simulink model "SuspensionModelBase"  (R2025b)
settings: Solver=ode23t  StartTime=0.0  StopTime=5  RelTol=1e-3
values from neighbouring files (symbols this model uses):
  car = get_suspension_default_params()    [run_suspension_standalone.m]
settings Model: Creator=91984  LastModifiedBy=91984

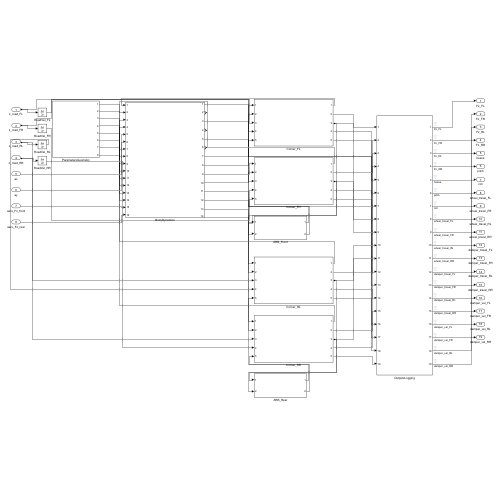
[thumbnail: Simulink's stored preview of the top-level diagram]
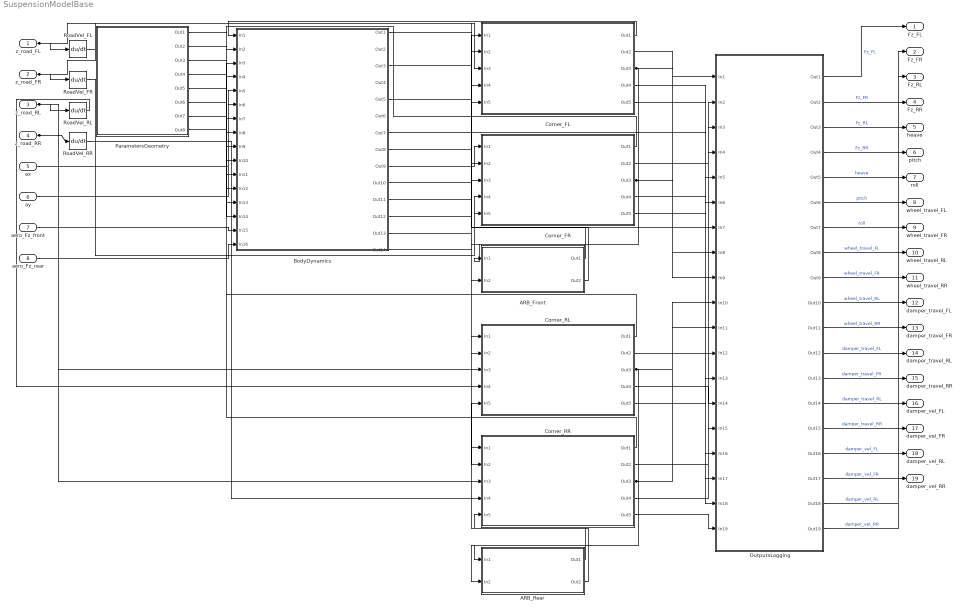
== system SuspensionModelBase ==
  z_road_FL : Inport
  z_road_FR : Inport  Port=2
  z_road_RL : Inport  Port=3
  z_road_RR : Inport  Port=4
  ax : Inport  Port=5
  ay : Inport  Port=6
  aero_Fz_front : Inport  Port=7
  aero_Fz_rear : Inport  Port=8
  ARB_Front : Subsystem
  ARB_Rear : Subsystem
  BodyDynamics : Subsystem
  Corner_FL : Subsystem
  Corner_FR : Subsystem
  Corner_RL : Subsystem
  Corner_RR : Subsystem
  OutputsLogging : Subsystem
  ParametersGeometry : Subsystem
  RoadVel_FL : Derivative
  RoadVel_FR : Derivative
  RoadVel_RL : Derivative
  RoadVel_RR : Derivative
  Fz_FL : Outport
  Fz_FR : Outport  Port=2
  Fz_RL : Outport  Port=3
  Fz_RR : Outport  Port=4
  heave : Outport  Port=5
  pitch : Outport  Port=6
  roll : Outport  Port=7
  wheel_travel_FL : Outport  Port=8
  wheel_travel_FR : Outport  Port=9
  wheel_travel_RL : Outport  Port=10
  wheel_travel_RR : Outport  Port=11
  damper_travel_FL : Outport  Port=12
  damper_travel_FR : Outport  Port=13
  damper_travel_RL : Outport  Port=14
  damper_travel_RR : Outport  Port=15
  damper_vel_FL : Outport  Port=16
  damper_vel_FR : Outport  Port=17
  damper_vel_RL : Outport  Port=18
  damper_vel_RR : Outport  Port=19
  wires:
  z_road_FL/1 -> RoadVel_FL/1, Corner_FL/3(In3)
  RoadVel_FL/1 -> Corner_FL/4(In4)
  z_road_FR/1 -> RoadVel_FR/1, Corner_FR/3(In3)
  RoadVel_FR/1 -> Corner_FR/4(In4)
  z_road_RL/1 -> RoadVel_RL/1, Corner_RL/3(In3)
  RoadVel_RL/1 -> Corner_RL/4(In4)
  z_road_RR/1 -> RoadVel_RR/1, Corner_RR/3(In3)
  RoadVel_RR/1 -> Corner_RR/4(In4)
  ax/1 -> BodyDynamics/5(In5)
  ay/1 -> BodyDynamics/6(In6)
  aero_Fz_front/1 -> BodyDynamics/15(In15)
  aero_Fz_rear/1 -> BodyDynamics/16(In16)
  ParametersGeometry/1(Out1) -> BodyDynamics/7(In7)
  ParametersGeometry/2(Out2) -> BodyDynamics/8(In8)
  ParametersGeometry/3(Out3) -> BodyDynamics/9(In9)
  ParametersGeometry/4(Out4) -> BodyDynamics/10(In10)
  ParametersGeometry/5(Out5) -> BodyDynamics/11(In11)
  ParametersGeometry/6(Out6) -> BodyDynamics/12(In12)
  ParametersGeometry/7(Out7) -> BodyDynamics/13(In13)
  ParametersGeometry/8(Out8) -> BodyDynamics/14(In14)
  BodyDynamics/7(Out7) -> Corner_FL/1(In1)
  BodyDynamics/8(Out8) -> Corner_FL/2(In2)
  BodyDynamics/9(Out9) -> Corner_FR/1(In1)
  BodyDynamics/10(Out10) -> Corner_FR/2(In2)
  BodyDynamics/11(Out11) -> Corner_RL/1(In1)
  BodyDynamics/12(Out12) -> Corner_RL/2(In2)
  BodyDynamics/13(Out13) -> Corner_RR/1(In1)
  BodyDynamics/14(Out14) -> Corner_RR/2(In2)
  Corner_FL/1(Out1) -> BodyDynamics/1(In1)
  Corner_FR/1(Out1) -> BodyDynamics/2(In2)
  Corner_RL/1(Out1) -> BodyDynamics/3(In3)
  Corner_RR/1(Out1) -> BodyDynamics/4(In4)
  Corner_FL/3(Out3) -> ARB_Front/1(In1), OutputsLogging/8(In8)
  Corner_FR/3(Out3) -> ARB_Front/2(In2), OutputsLogging/9(In9)
  ARB_Front/1(Out1) -> Corner_FL/5(In5)
  ARB_Front/2(Out2) -> Corner_FR/5(In5)
  Corner_RL/3(Out3) -> ARB_Rear/1(In1), OutputsLogging/10(In10)
  Corner_RR/3(Out3) -> ARB_Rear/2(In2), OutputsLogging/11(In11)
  ARB_Rear/1(Out1) -> Corner_RL/5(In5)
  ARB_Rear/2(Out2) -> Corner_RR/5(In5)
  Corner_FL/2(Out2) -> OutputsLogging/1(In1)
  Corner_FR/2(Out2) -> OutputsLogging/2(In2)
  Corner_RL/2(Out2) -> OutputsLogging/3(In3)
  Corner_RR/2(Out2) -> OutputsLogging/4(In4)
  BodyDynamics/1(Out1) -> OutputsLogging/5(In5)
  BodyDynamics/3(Out3) -> OutputsLogging/6(In6)
  BodyDynamics/5(Out5) -> OutputsLogging/7(In7)
  Corner_FL/4(Out4) -> OutputsLogging/12(In12)
  Corner_FR/4(Out4) -> OutputsLogging/13(In13)
  Corner_RL/4(Out4) -> OutputsLogging/14(In14)
  Corner_RR/4(Out4) -> OutputsLogging/15(In15)
  Corner_FL/5(Out5) -> OutputsLogging/16(In16)
  Corner_FR/5(Out5) -> OutputsLogging/17(In17)
  Corner_RL/5(Out5) -> OutputsLogging/18(In18)
  Corner_RR/5(Out5) -> OutputsLogging/19(In19)
  OutputsLogging/1(Out1) -> Fz_FL/1  "Fz_FL"
  OutputsLogging/2(Out2) -> Fz_FR/1  "Fz_FR"
  OutputsLogging/3(Out3) -> Fz_RL/1  "Fz_RL"
  OutputsLogging/4(Out4) -> Fz_RR/1  "Fz_RR"
  OutputsLogging/5(Out5) -> heave/1  "heave"
  OutputsLogging/6(Out6) -> pitch/1  "pitch"
  OutputsLogging/7(Out7) -> roll/1  "roll"
  OutputsLogging/8(Out8) -> wheel_travel_FL/1  "wheel_travel_FL"
  OutputsLogging/9(Out9) -> wheel_travel_FR/1  "wheel_travel_FR"
  OutputsLogging/10(Out10) -> wheel_travel_RL/1  "wheel_travel_RL"
  OutputsLogging/11(Out11) -> wheel_travel_RR/1  "wheel_travel_RR"
  OutputsLogging/12(Out12) -> damper_travel_FL/1  "damper_travel_FL"
  OutputsLogging/13(Out13) -> damper_travel_FR/1  "damper_travel_FR"
  OutputsLogging/14(Out14) -> damper_travel_RL/1  "damper_travel_RL"
  OutputsLogging/15(Out15) -> damper_travel_RR/1  "damper_travel_RR"
  OutputsLogging/16(Out16) -> damper_vel_FL/1  "damper_vel_FL"
  OutputsLogging/17(Out17) -> damper_vel_FR/1  "damper_vel_FR"
  OutputsLogging/18(Out18) -> damper_vel_RL/1  "damper_vel_RL"
  OutputsLogging/19(Out19) -> damper_vel_RR/1  "damper_vel_RR"

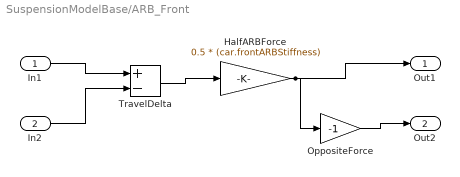
== system SuspensionModelBase/ARB_Front ==
  In1 : Inport
  In2 : Inport  Port=2
  HalfARBForce : Gain  Gain=0.5 * (car.frontARBStiffness)
  OppositeForce : Gain  Gain=-1
  TravelDelta : Sum  Inputs=+-
  Out1 : Outport
  Out2 : Outport  Port=2
  wires:
  In1/1 -> TravelDelta/1
  In2/1 -> TravelDelta/2
  TravelDelta/1 -> HalfARBForce/1
  HalfARBForce/1 -> Out1/1, OppositeForce/1
  OppositeForce/1 -> Out2/1

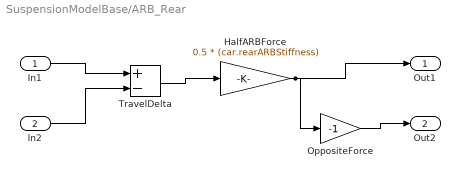
== system SuspensionModelBase/ARB_Rear ==
  In1 : Inport
  In2 : Inport  Port=2
  HalfARBForce : Gain  Gain=0.5 * (car.rearARBStiffness)
  OppositeForce : Gain  Gain=-1
  TravelDelta : Sum  Inputs=+-
  Out1 : Outport
  Out2 : Outport  Port=2
  wires:
  In1/1 -> TravelDelta/1
  In2/1 -> TravelDelta/2
  TravelDelta/1 -> HalfARBForce/1
  HalfARBForce/1 -> Out1/1, OppositeForce/1
  OppositeForce/1 -> Out2/1

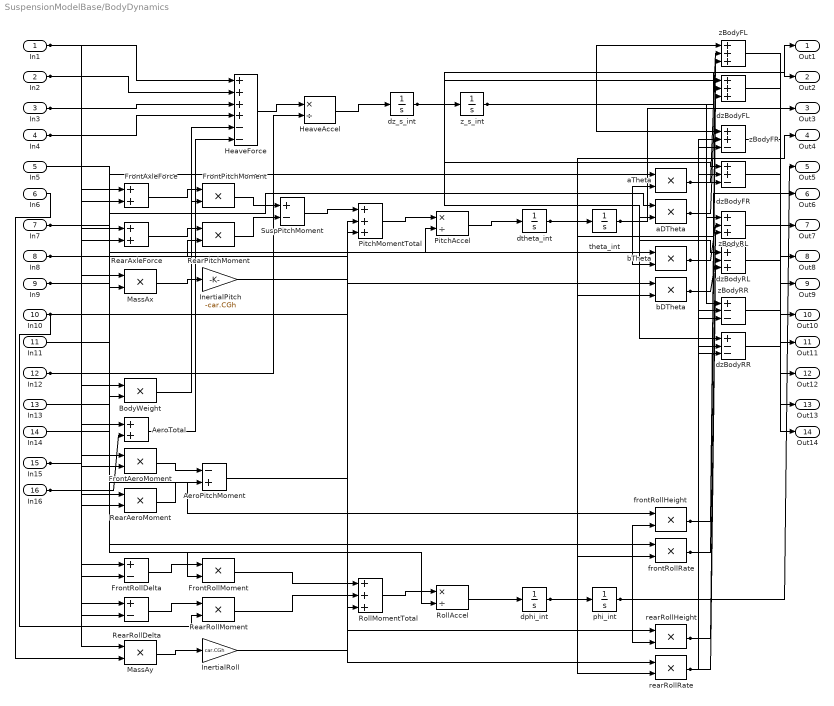
== system SuspensionModelBase/BodyDynamics ==
  In1 : Inport
  In2 : Inport  Port=2
  In3 : Inport  Port=3
  In4 : Inport  Port=4
  In5 : Inport  Port=5
  In6 : Inport  Port=6
  In7 : Inport  Port=7
  In8 : Inport  Port=8
  In9 : Inport  Port=9
  In10 : Inport  Port=10
  In11 : Inport  Port=11
  In12 : Inport  Port=12
  In13 : Inport  Port=13
  In14 : Inport  Port=14
  In15 : Inport  Port=15
  In16 : Inport  Port=16
  AeroPitchMoment : Sum  Inputs=-+
  AeroTotal : Sum
  BodyWeight : Product  Inputs=**
  FrontAeroMoment : Product  Inputs=**
  FrontAxleForce : Sum
  FrontPitchMoment : Product  Inputs=**
  FrontRollDelta : Sum  Inputs=+-
  FrontRollMoment : Product  Inputs=**
  HeaveAccel : Product  Inputs=*/
  HeaveForce : Sum  Inputs=++++--
  InertialPitch : Gain  Gain=-car.CGh
  InertialRoll : Gain  Gain=car.CGh
  MassAx : Product  Inputs=**
  MassAy : Product  Inputs=**
  PitchAccel : Product  Inputs=*/
  PitchMomentTotal : Sum  Inputs=+++
  RearAeroMoment : Product  Inputs=**
  RearAxleForce : Sum
  RearPitchMoment : Product  Inputs=**
  RearRollDelta : Sum  Inputs=+-
  RearRollMoment : Product  Inputs=**
  RollAccel : Product  Inputs=*/
  RollMomentTotal : Sum  Inputs=+++
  SuspPitchMoment : Sum  Inputs=+-
  aDTheta : Product  Inputs=**
  aTheta : Product  Inputs=**
  bDTheta : Product  Inputs=**
  bTheta : Product  Inputs=**
  dphi_int : Integrator
  dtheta_int : Integrator
  dzBodyFL : Sum  Inputs=+++
  dzBodyFR : Sum  Inputs=++-
  dzBodyRL : Sum  Inputs=+-+
  dzBodyRR : Sum  Inputs=+--
  dz_s_int : Integrator
  frontRollHeight : Product  Inputs=**
  frontRollRate : Product  Inputs=**
  phi_int : Integrator
  rearRollHeight : Product  Inputs=**
  rearRollRate : Product  Inputs=**
  theta_int : Integrator
  zBodyFL : Sum  Inputs=+++
  zBodyFR : Sum  Inputs=++-
  zBodyRL : Sum  Inputs=+-+
  zBodyRR : Sum  Inputs=+--
  z_s_int : Integrator
  Out1 : Outport
  Out2 : Outport  Port=2
  Out3 : Outport  Port=3
  Out4 : Outport  Port=4
  Out5 : Outport  Port=5
  Out6 : Outport  Port=6
  Out7 : Outport  Port=7
  Out8 : Outport  Port=8
  Out9 : Outport  Port=9
  Out10 : Outport  Port=10
  Out11 : Outport  Port=11
  Out12 : Outport  Port=12
  Out13 : Outport  Port=13
  Out14 : Outport  Port=14
  wires:
  In1/1 -> HeaveForce/1, FrontAxleForce/1, FrontRollDelta/1
  In2/1 -> HeaveForce/2, FrontAxleForce/2, FrontRollDelta/2
  In3/1 -> HeaveForce/3, RearAxleForce/1, RearRollDelta/1
  In4/1 -> HeaveForce/4, RearAxleForce/2, RearRollDelta/2
  In12/1 -> BodyWeight/1, HeaveAccel/2, MassAx/1, MassAy/1
  In11/1 -> BodyWeight/2
  BodyWeight/1 -> HeaveForce/5
  In15/1 -> AeroTotal/1, FrontAeroMoment/1
  In16/1 -> AeroTotal/2, RearAeroMoment/1
  AeroTotal/1 -> HeaveForce/6
  HeaveForce/1 -> HeaveAccel/1
  HeaveAccel/1 -> dz_s_int/1
  dz_s_int/1 -> z_s_int/1, Out2/1, dzBodyFL/1, dzBodyFR/1, dzBodyRL/1, dzBodyRR/1
  z_s_int/1 -> Out1/1, zBodyFL/1, zBodyFR/1, zBodyRL/1, zBodyRR/1
  FrontAxleForce/1 -> FrontPitchMoment/1
  In7/1 -> FrontPitchMoment/2, FrontAeroMoment/2, aTheta/1, aDTheta/1
  RearAxleForce/1 -> RearPitchMoment/1
  In8/1 -> RearPitchMoment/2, RearAeroMoment/2, bTheta/1, bDTheta/1
  FrontPitchMoment/1 -> SuspPitchMoment/1
  RearPitchMoment/1 -> SuspPitchMoment/2
  In5/1 -> MassAx/2
  MassAx/1 -> InertialPitch/1
  FrontAeroMoment/1 -> AeroPitchMoment/1
  RearAeroMoment/1 -> AeroPitchMoment/2
  SuspPitchMoment/1 -> PitchMomentTotal/1
  InertialPitch/1 -> PitchMomentTotal/2
  AeroPitchMoment/1 -> PitchMomentTotal/3
  PitchMomentTotal/1 -> PitchAccel/1
  In13/1 -> PitchAccel/2
  PitchAccel/1 -> dtheta_int/1
  dtheta_int/1 -> theta_int/1, Out4/1, aDTheta/2, bDTheta/2
  theta_int/1 -> Out3/1, aTheta/2, bTheta/2
  FrontRollDelta/1 -> FrontRollMoment/1
  In9/1 -> FrontRollMoment/2, frontRollHeight/1, frontRollRate/1
  RearRollDelta/1 -> RearRollMoment/1
  In10/1 -> RearRollMoment/2, rearRollHeight/1, rearRollRate/1
  In6/1 -> MassAy/2
  MassAy/1 -> InertialRoll/1
  FrontRollMoment/1 -> RollMomentTotal/1
  RearRollMoment/1 -> RollMomentTotal/2
  InertialRoll/1 -> RollMomentTotal/3
  RollMomentTotal/1 -> RollAccel/1
  In14/1 -> RollAccel/2
  RollAccel/1 -> dphi_int/1
  dphi_int/1 -> phi_int/1, Out6/1, frontRollRate/2, rearRollRate/2
  phi_int/1 -> Out5/1, frontRollHeight/2, rearRollHeight/2
  aTheta/1 -> zBodyFL/2, zBodyFR/2
  frontRollHeight/1 -> zBodyFL/3, zBodyFR/3
  zBodyFL/1 -> Out7/1
  aDTheta/1 -> dzBodyFL/2, dzBodyFR/2
  frontRollRate/1 -> dzBodyFL/3, dzBodyFR/3
  dzBodyFL/1 -> Out8/1
  zBodyFR/1 -> Out9/1
  dzBodyFR/1 -> Out10/1
  bTheta/1 -> zBodyRL/2, zBodyRR/2
  rearRollHeight/1 -> zBodyRL/3, zBodyRR/3
  zBodyRL/1 -> Out11/1
  bDTheta/1 -> dzBodyRL/2, dzBodyRR/2
  rearRollRate/1 -> dzBodyRL/3, dzBodyRR/3
  dzBodyRL/1 -> Out12/1
  zBodyRR/1 -> Out13/1
  dzBodyRR/1 -> Out14/1

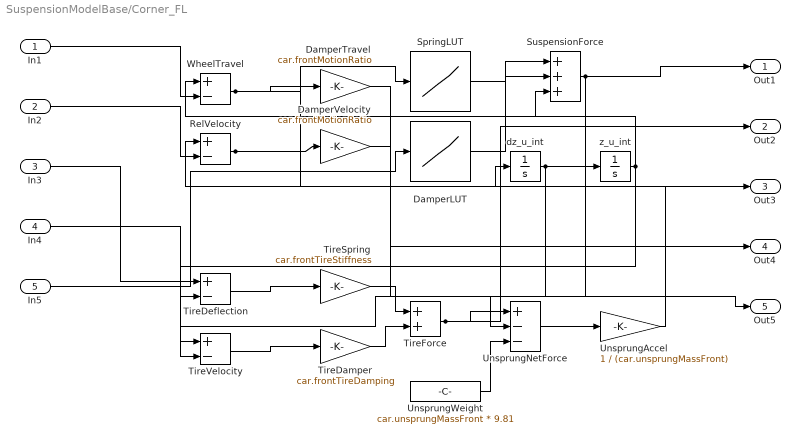
== system SuspensionModelBase/Corner_FL ==
  In1 : Inport
  In2 : Inport  Port=2
  In3 : Inport  Port=3
  In4 : Inport  Port=4
  In5 : Inport  Port=5
  DamperLUT : Lookup_n-D  NumberOfTableDimensions=1  BreakpointsForDimension1=curves.front.damper.x  Table=curves.front.damper.y  ExtrapMethod=Clip  InternalRulePriority=Speed  RndMeth=Simplest
  DamperTravel : Gain  Gain=car.frontMotionRatio
  DamperVelocity : Gain  Gain=car.frontMotionRatio
  RelVelocity : Sum  Inputs=+-
  SpringLUT : Lookup_n-D  NumberOfTableDimensions=1  BreakpointsForDimension1=curves.front.spring.x  Table=curves.front.spring.y  ExtrapMethod=Clip  InternalRulePriority=Speed  RndMeth=Simplest
  SuspensionForce : Sum  Inputs=+++
  TireDamper : Gain  Gain=car.frontTireDamping
  TireDeflection : Sum  Inputs=+-
  TireForce : Sum
  TireSpring : Gain  Gain=car.frontTireStiffness
  TireVelocity : Sum  Inputs=+-
  UnsprungAccel : Gain  Gain=1 / (car.unsprungMassFront)
  UnsprungNetForce : Sum  Inputs=+--
  UnsprungWeight : Constant  Value=car.unsprungMassFront * 9.81
  WheelTravel : Sum  Inputs=+-
  dz_u_int : Integrator
  z_u_int : Integrator
  Out1 : Outport
  Out2 : Outport  Port=2
  Out3 : Outport  Port=3
  Out4 : Outport  Port=4
  Out5 : Outport  Port=5
  wires:
  z_u_int/1 -> WheelTravel/1, TireDeflection/2
  In1/1 -> WheelTravel/2
  WheelTravel/1 -> DamperTravel/1, SpringLUT/1, Out3/1
  DamperTravel/1 -> Out4/1
  dz_u_int/1 -> RelVelocity/1, TireVelocity/2, z_u_int/1
  In2/1 -> RelVelocity/2
  RelVelocity/1 -> DamperVelocity/1, DamperLUT/1
  DamperVelocity/1 -> Out5/1
  SpringLUT/1 -> SuspensionForce/1
  DamperLUT/1 -> SuspensionForce/2
  In5/1 -> SuspensionForce/3
  SuspensionForce/1 -> Out1/1, UnsprungNetForce/2
  In3/1 -> TireDeflection/1
  TireDeflection/1 -> TireSpring/1
  In4/1 -> TireVelocity/1
  TireVelocity/1 -> TireDamper/1
  TireSpring/1 -> TireForce/1
  TireDamper/1 -> TireForce/2
  TireForce/1 -> Out2/1, UnsprungNetForce/1
  UnsprungWeight/1 -> UnsprungNetForce/3
  UnsprungNetForce/1 -> UnsprungAccel/1
  UnsprungAccel/1 -> dz_u_int/1

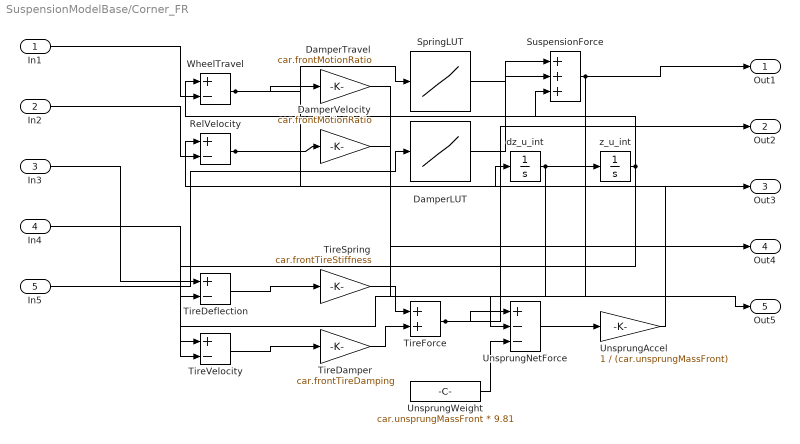
== system SuspensionModelBase/Corner_FR ==
  In1 : Inport
  In2 : Inport  Port=2
  In3 : Inport  Port=3
  In4 : Inport  Port=4
  In5 : Inport  Port=5
  DamperLUT : Lookup_n-D  NumberOfTableDimensions=1  BreakpointsForDimension1=curves.front.damper.x  Table=curves.front.damper.y  ExtrapMethod=Clip  InternalRulePriority=Speed  RndMeth=Simplest
  DamperTravel : Gain  Gain=car.frontMotionRatio
  DamperVelocity : Gain  Gain=car.frontMotionRatio
  RelVelocity : Sum  Inputs=+-
  SpringLUT : Lookup_n-D  NumberOfTableDimensions=1  BreakpointsForDimension1=curves.front.spring.x  Table=curves.front.spring.y  ExtrapMethod=Clip  InternalRulePriority=Speed  RndMeth=Simplest
  SuspensionForce : Sum  Inputs=+++
  TireDamper : Gain  Gain=car.frontTireDamping
  TireDeflection : Sum  Inputs=+-
  TireForce : Sum
  TireSpring : Gain  Gain=car.frontTireStiffness
  TireVelocity : Sum  Inputs=+-
  UnsprungAccel : Gain  Gain=1 / (car.unsprungMassFront)
  UnsprungNetForce : Sum  Inputs=+--
  UnsprungWeight : Constant  Value=car.unsprungMassFront * 9.81
  WheelTravel : Sum  Inputs=+-
  dz_u_int : Integrator
  z_u_int : Integrator
  Out1 : Outport
  Out2 : Outport  Port=2
  Out3 : Outport  Port=3
  Out4 : Outport  Port=4
  Out5 : Outport  Port=5
  wires:
  z_u_int/1 -> WheelTravel/1, TireDeflection/2
  In1/1 -> WheelTravel/2
  WheelTravel/1 -> DamperTravel/1, SpringLUT/1, Out3/1
  DamperTravel/1 -> Out4/1
  dz_u_int/1 -> RelVelocity/1, TireVelocity/2, z_u_int/1
  In2/1 -> RelVelocity/2
  RelVelocity/1 -> DamperVelocity/1, DamperLUT/1
  DamperVelocity/1 -> Out5/1
  SpringLUT/1 -> SuspensionForce/1
  DamperLUT/1 -> SuspensionForce/2
  In5/1 -> SuspensionForce/3
  SuspensionForce/1 -> Out1/1, UnsprungNetForce/2
  In3/1 -> TireDeflection/1
  TireDeflection/1 -> TireSpring/1
  In4/1 -> TireVelocity/1
  TireVelocity/1 -> TireDamper/1
  TireSpring/1 -> TireForce/1
  TireDamper/1 -> TireForce/2
  TireForce/1 -> Out2/1, UnsprungNetForce/1
  UnsprungWeight/1 -> UnsprungNetForce/3
  UnsprungNetForce/1 -> UnsprungAccel/1
  UnsprungAccel/1 -> dz_u_int/1

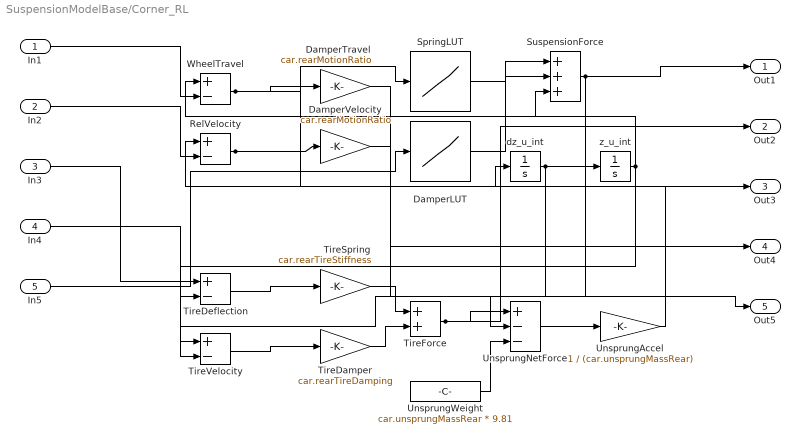
== system SuspensionModelBase/Corner_RL ==
  In1 : Inport
  In2 : Inport  Port=2
  In3 : Inport  Port=3
  In4 : Inport  Port=4
  In5 : Inport  Port=5
  DamperLUT : Lookup_n-D  NumberOfTableDimensions=1  BreakpointsForDimension1=curves.rear.damper.x  Table=curves.rear.damper.y  ExtrapMethod=Clip  InternalRulePriority=Speed  RndMeth=Simplest
  DamperTravel : Gain  Gain=car.rearMotionRatio
  DamperVelocity : Gain  Gain=car.rearMotionRatio
  RelVelocity : Sum  Inputs=+-
  SpringLUT : Lookup_n-D  NumberOfTableDimensions=1  BreakpointsForDimension1=curves.rear.spring.x  Table=curves.rear.spring.y  ExtrapMethod=Clip  InternalRulePriority=Speed  RndMeth=Simplest
  SuspensionForce : Sum  Inputs=+++
  TireDamper : Gain  Gain=car.rearTireDamping
  TireDeflection : Sum  Inputs=+-
  TireForce : Sum
  TireSpring : Gain  Gain=car.rearTireStiffness
  TireVelocity : Sum  Inputs=+-
  UnsprungAccel : Gain  Gain=1 / (car.unsprungMassRear)
  UnsprungNetForce : Sum  Inputs=+--
  UnsprungWeight : Constant  Value=car.unsprungMassRear * 9.81
  WheelTravel : Sum  Inputs=+-
  dz_u_int : Integrator
  z_u_int : Integrator
  Out1 : Outport
  Out2 : Outport  Port=2
  Out3 : Outport  Port=3
  Out4 : Outport  Port=4
  Out5 : Outport  Port=5
  wires:
  z_u_int/1 -> WheelTravel/1, TireDeflection/2
  In1/1 -> WheelTravel/2
  WheelTravel/1 -> DamperTravel/1, SpringLUT/1, Out3/1
  DamperTravel/1 -> Out4/1
  dz_u_int/1 -> RelVelocity/1, TireVelocity/2, z_u_int/1
  In2/1 -> RelVelocity/2
  RelVelocity/1 -> DamperVelocity/1, DamperLUT/1
  DamperVelocity/1 -> Out5/1
  SpringLUT/1 -> SuspensionForce/1
  DamperLUT/1 -> SuspensionForce/2
  In5/1 -> SuspensionForce/3
  SuspensionForce/1 -> Out1/1, UnsprungNetForce/2
  In3/1 -> TireDeflection/1
  TireDeflection/1 -> TireSpring/1
  In4/1 -> TireVelocity/1
  TireVelocity/1 -> TireDamper/1
  TireSpring/1 -> TireForce/1
  TireDamper/1 -> TireForce/2
  TireForce/1 -> Out2/1, UnsprungNetForce/1
  UnsprungWeight/1 -> UnsprungNetForce/3
  UnsprungNetForce/1 -> UnsprungAccel/1
  UnsprungAccel/1 -> dz_u_int/1

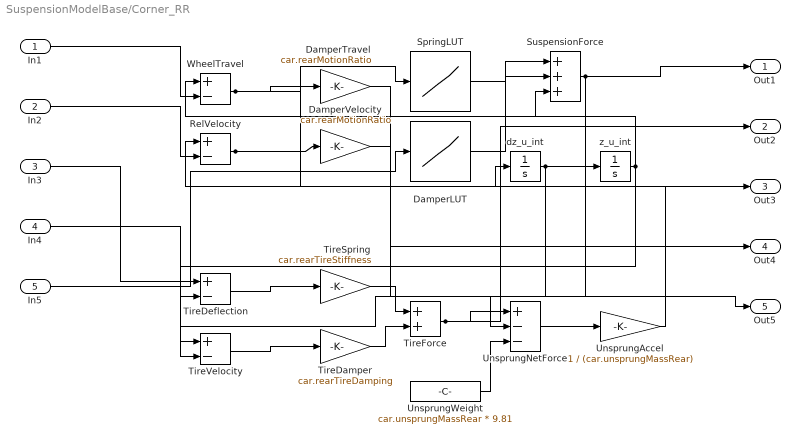
== system SuspensionModelBase/Corner_RR ==
  In1 : Inport
  In2 : Inport  Port=2
  In3 : Inport  Port=3
  In4 : Inport  Port=4
  In5 : Inport  Port=5
  DamperLUT : Lookup_n-D  NumberOfTableDimensions=1  BreakpointsForDimension1=curves.rear.damper.x  Table=curves.rear.damper.y  ExtrapMethod=Clip  InternalRulePriority=Speed  RndMeth=Simplest
  DamperTravel : Gain  Gain=car.rearMotionRatio
  DamperVelocity : Gain  Gain=car.rearMotionRatio
  RelVelocity : Sum  Inputs=+-
  SpringLUT : Lookup_n-D  NumberOfTableDimensions=1  BreakpointsForDimension1=curves.rear.spring.x  Table=curves.rear.spring.y  ExtrapMethod=Clip  InternalRulePriority=Speed  RndMeth=Simplest
  SuspensionForce : Sum  Inputs=+++
  TireDamper : Gain  Gain=car.rearTireDamping
  TireDeflection : Sum  Inputs=+-
  TireForce : Sum
  TireSpring : Gain  Gain=car.rearTireStiffness
  TireVelocity : Sum  Inputs=+-
  UnsprungAccel : Gain  Gain=1 / (car.unsprungMassRear)
  UnsprungNetForce : Sum  Inputs=+--
  UnsprungWeight : Constant  Value=car.unsprungMassRear * 9.81
  WheelTravel : Sum  Inputs=+-
  dz_u_int : Integrator
  z_u_int : Integrator
  Out1 : Outport
  Out2 : Outport  Port=2
  Out3 : Outport  Port=3
  Out4 : Outport  Port=4
  Out5 : Outport  Port=5
  wires:
  z_u_int/1 -> WheelTravel/1, TireDeflection/2
  In1/1 -> WheelTravel/2
  WheelTravel/1 -> DamperTravel/1, SpringLUT/1, Out3/1
  DamperTravel/1 -> Out4/1
  dz_u_int/1 -> RelVelocity/1, TireVelocity/2, z_u_int/1
  In2/1 -> RelVelocity/2
  RelVelocity/1 -> DamperVelocity/1, DamperLUT/1
  DamperVelocity/1 -> Out5/1
  SpringLUT/1 -> SuspensionForce/1
  DamperLUT/1 -> SuspensionForce/2
  In5/1 -> SuspensionForce/3
  SuspensionForce/1 -> Out1/1, UnsprungNetForce/2
  In3/1 -> TireDeflection/1
  TireDeflection/1 -> TireSpring/1
  In4/1 -> TireVelocity/1
  TireVelocity/1 -> TireDamper/1
  TireSpring/1 -> TireForce/1
  TireDamper/1 -> TireForce/2
  TireForce/1 -> Out2/1, UnsprungNetForce/1
  UnsprungWeight/1 -> UnsprungNetForce/3
  UnsprungNetForce/1 -> UnsprungAccel/1
  UnsprungAccel/1 -> dz_u_int/1

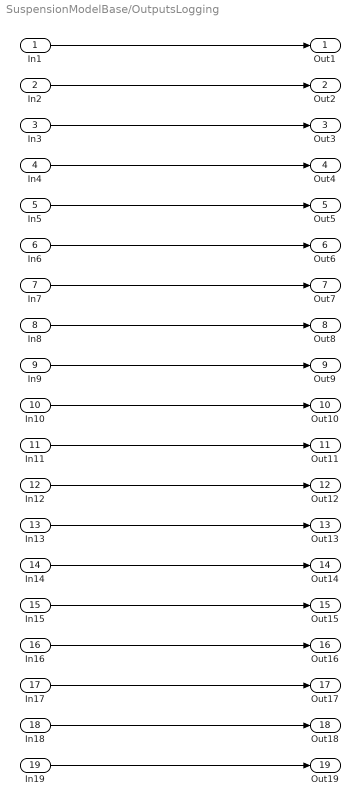
== system SuspensionModelBase/OutputsLogging ==
  In1 : Inport
  In2 : Inport  Port=2
  In3 : Inport  Port=3
  In4 : Inport  Port=4
  In5 : Inport  Port=5
  In6 : Inport  Port=6
  In7 : Inport  Port=7
  In8 : Inport  Port=8
  In9 : Inport  Port=9
  In10 : Inport  Port=10
  In11 : Inport  Port=11
  In12 : Inport  Port=12
  In13 : Inport  Port=13
  In14 : Inport  Port=14
  In15 : Inport  Port=15
  In16 : Inport  Port=16
  In17 : Inport  Port=17
  In18 : Inport  Port=18
  In19 : Inport  Port=19
  Out1 : Outport
  Out2 : Outport  Port=2
  Out3 : Outport  Port=3
  Out4 : Outport  Port=4
  Out5 : Outport  Port=5
  Out6 : Outport  Port=6
  Out7 : Outport  Port=7
  Out8 : Outport  Port=8
  Out9 : Outport  Port=9
  Out10 : Outport  Port=10
  Out11 : Outport  Port=11
  Out12 : Outport  Port=12
  Out13 : Outport  Port=13
  Out14 : Outport  Port=14
  Out15 : Outport  Port=15
  Out16 : Outport  Port=16
  Out17 : Outport  Port=17
  Out18 : Outport  Port=18
  Out19 : Outport  Port=19
  wires:
  In1/1 -> Out1/1
  In2/1 -> Out2/1
  In3/1 -> Out3/1
  In4/1 -> Out4/1
  In5/1 -> Out5/1
  In6/1 -> Out6/1
  In7/1 -> Out7/1
  In8/1 -> Out8/1
  In9/1 -> Out9/1
  In10/1 -> Out10/1
  In11/1 -> Out11/1
  In12/1 -> Out12/1
  In13/1 -> Out13/1
  In14/1 -> Out14/1
  In15/1 -> Out15/1
  In16/1 -> Out16/1
  In17/1 -> Out17/1
  In18/1 -> Out18/1
  In19/1 -> Out19/1

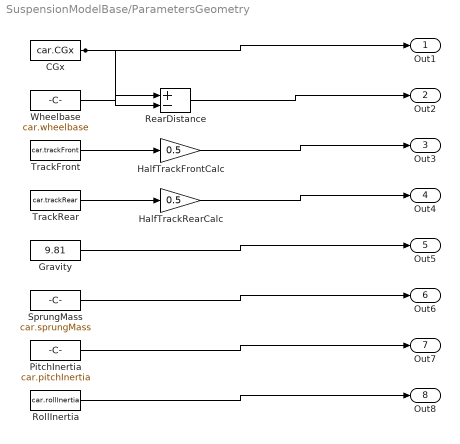
== system SuspensionModelBase/ParametersGeometry ==
  CGx : Constant  Value=car.CGx
  Gravity : Constant  Value=9.81
  HalfTrackFrontCalc : Gain  Gain=0.5
  HalfTrackRearCalc : Gain  Gain=0.5
  PitchInertia : Constant  Value=car.pitchInertia
  RearDistance : Sum  Inputs=+-
  RollInertia : Constant  Value=car.rollInertia
  SprungMass : Constant  Value=car.sprungMass
  TrackFront : Constant  Value=car.trackFront
  TrackRear : Constant  Value=car.trackRear
  Wheelbase : Constant  Value=car.wheelbase
  Out1 : Outport
  Out2 : Outport  Port=2
  Out3 : Outport  Port=3
  Out4 : Outport  Port=4
  Out5 : Outport  Port=5
  Out6 : Outport  Port=6
  Out7 : Outport  Port=7
  Out8 : Outport  Port=8
  wires:
  CGx/1 -> Out1/1, RearDistance/2
  Wheelbase/1 -> RearDistance/1
  RearDistance/1 -> Out2/1
  TrackFront/1 -> HalfTrackFrontCalc/1
  HalfTrackFrontCalc/1 -> Out3/1
  TrackRear/1 -> HalfTrackRearCalc/1
  HalfTrackRearCalc/1 -> Out4/1
  Gravity/1 -> Out5/1
  SprungMass/1 -> Out6/1
  PitchInertia/1 -> Out7/1
  RollInertia/1 -> Out8/1
